simulink model "slexVariantSourceAndSink_org"  (Simulink 10.0)
settings: Solver=FixedStepAuto  StartTime=0.0  StopTime=10.0  RelTol=1e-3  EnableMultiTasking=on
PreLoadFcn:
  | addpath(fileparts(which(bdroot)));
PostLoadFcn:
  | V = Simulink.Parameter(int32(1));
  | V.StorageClass = 'Define (Custom)';
  | V.CoderInfo.CustomAttributes.HeaderFile='variant_defines.h';
  | 
  | W=copy(V);
libraries: simulink x1
settings Model: Creator=The MathWorks, Inc.  LastModifiedBy=bhisma
settings DataIOCC: LimitDataPoints=on  OutputSaveName=out1,out2,out3
settings OptimizationCC: LifeSpan=1  EfficientTunableParamExpr=on
settings DebuggingCC: UnderspecifiedInitializationDetection=Simplified  MergeDetectMultiDrivingBlocksExec=error  ParameterPrecisionLossMsg=none  AllowSymbolicDim=off
settings SFSimCC: MATLABDynamicMemAlloc=off
settings RTWCC: Description=Embedded Coder  SystemTargetFile=ert.tlc  TemplateMakefile=ert_default_tmf
settings CodeAppCC: IgnoreCustomStorageClasses=off  CustomSymbolStrModelFcn=$N
settings ERTTargetCC: MultiwordLength=2048  GenerateSampleERTMain=on  ERTCustomFileTemplate=example_file_process.tlc  ConvertIfToSwitch=off  SuppressUnreachableDefaultCases=off
settings ConfigComp: CovExternalEMLEnable=off

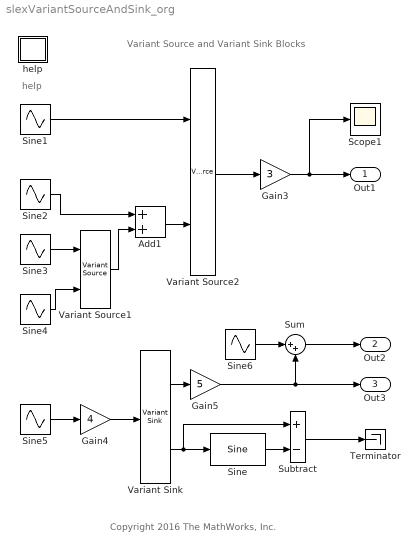
== system slexVariantSourceAndSink_org ==
  note: Variant Source and Variant Sink Blocks
  note: Copyright 2016 The MathWorks, Inc.
  note: help
  Add1 : Sum
  Gain3 : Gain  Gain=3
  Gain4 : Gain  Gain=4
  Gain5 : Gain  Gain=5
  Scope1 : Scope
  Sine : simulink/Lookup Tables/Sine  Formula=sin(2*pi*u)  NumDataPoints=(2^5)+1  OutputWordLength=16  InternalRulePriority=Speed
      settings: SourceProductName=Simulink
  Sine{1..6} (6 alike) : Sin  SineType=Sample based  SampleTime=0.2
  Subtract : Sum  Inputs=+-
  Sum : Sum  Inputs=|++
  Terminator : Terminator
  Variant Sink : VariantSink  VariantControls=DataTag0
      settings: GeneratePreprocessorConditionals=on
  Variant Source1 : VariantSource  VariantControls=DataTag1
  Variant Source2 : VariantSource  VariantControls=DataTag2
      settings: GeneratePreprocessorConditionals=on  AllowZeroVariantControls=on
  help : Subsystem
      mask Display: disp('?')
  Out1 : Outport  VectorParamsAs1DForOutWhenUnconnected=off
  Out2 : Outport  Port=2  VectorParamsAs1DForOutWhenUnconnected=off
  Out3 : Outport  Port=3  VectorParamsAs1DForOutWhenUnconnected=off
  wires:
  Sine1/1 -> Variant Source2/1
  Add1/1 -> Variant Source2/2
  Sine2/1 -> Add1/1
  Variant Source2/1 -> Gain3/1
  Gain3/1 -> Scope1/1, Out1/1
  Gain4/1 -> Variant Sink/1
  Sine5/1 -> Gain4/1
  Sum/1 -> Out2/1
  Variant Sink/1 -> Gain5/1
  Sine6/1 -> Sum/1
  Sine3/1 -> Variant Source1/1
  Sine4/1 -> Variant Source1/2
  Variant Source1/1 -> Add1/2
  Variant Sink/2 -> Subtract/1, Sine/1
  Subtract/1 -> Terminator/1
  Sine/1 -> Subtract/2
  Gain5/1 -> Out3/1, Sum/2

== system slexVariantSourceAndSink_org/help ==
  note: This illustrates how the Variant Source and Sink blocks define variant choice regions based on block connectivity. The variant regions are computed by Simulink when you run " Simulation -> Update Diagram ". The process of computing the variant choice regions is called variant condition propagation. The Variant Source provides variation on the source of a signal and the Variant Sink block provides variation on the destination (sink) of a signal. You can select "Display > Blocks > Variant Conditions" to view the variant condition annotations with a legend as described below.
      |
      | For example, Variant Source1 has conditions W==1 and W==2 for its input ports. W is a variant control variable and is defined in the PostLoadFcn of "File -> Model Properties -> Callbacks". The Sine3 block is active when W==1 and the Sine4 block is active when W==2. Examining the Variant Source2 block, we have the first input port active when V==1 and the second input port active when V==2. The Add1 block is active when V==2 and the propagation continues, when means the Variant Source1 is active when V==2, likewise the Sine3 and Sine4 can only be active when V==2, therefore the Sine3 is assigned the variant condition V==2 && W==1 and the Sine4 is assigned V==2 && W==2.
      |
      | If we select the " Allow zero active variant controls " on the Variant Source2 block parameter dialog , then the Gain3, Scope1, and Out1 will be assigned the variant condition, "V==1 || V==2".
      |
      | The Variant Sink specifies conditions W==1 and W==2 for its output ports. These conditions are propagated forward to the connected blocks. The Gain5 block is assigned the condition, W==1. The Sum block illustrates two key concepts in variant condition propagation:
      | Signals are only variant if explicitly marked or when all paths can be proven to be variant. To make the Sine6, Sum, Out2 variant you need to place a Single-Input Single-Output Variant Source before Out2 (or after Sine6)
      | Reading an inactive signal is equivalent to reading "ground". When W ~= 1, then the bottom input to the Sum block is inactive and Out2 = Sine6 + ground.
      |
      | The second output port of the Variant Sink block has the condition W==2 and this is propagated forward to the Sine, Subtract, and Out4 blocks. If you select " Allow zero active variant controls " on the Variant Sink block parameter dialog , then the Sine5 and Gain4 will be assigned the variant condition W==2.
      |
      | The Variant Source and Variant Sink block have the 'Analyze all choices during update diagram and generate preprocessor conditionals" parameter selected. This means that the generated code from the Simulink Embedded Coder will have #if COND present in the generated code and you select the active choice at code compile-time. If you unselect this parameter, then the generated code will have only the active choice present.
      |
      | Legend
      |
      | To view variant condition annotations for this model, from the Simulink editor menu, select
      | "Display > Blocks > Variant Conditions".
      | If it is already selected, you can run Updated Diagram (^D) to compile the model and display the conditions. There is also a separate Variant Condition legend window.
      | The Variant Condition legend displays on the block " v:C " where C represents the variant condition index on the legend.
      | There are no annotations on unconditional blocks.
      | The v:C labels in the legend are hyper-linked and highlight the blocks with condition, C.
      | The condition in the Description field of the annotation wraps (uses multiple lines when it is long).
      | The table shows the final propagated (computed) conditions for blocks. For example, conditions that you entered in Variant Source blocks may or may not appear in the table. They will only appear in the table if the condition was actually applied to a block. This reduces clutter in the legend.
      | The conditions in the table are sorted.
      | Conditions will be false if the Simulink variant condition expression engine can prove the blocks will never run. For example, Sine4 feeds the 2nd input of Variant Source1. If we change the condition of the 2nd input port on the Variant Source1 dialog, from W==2 to V==4 , this will result in the condition V==4 && V==2 for Sine4 which is always false. This condition arises because the Variant Source1 feeds the Add1 block which is connected to the 2nd input of Variant Source2, which says Variant Source1 will only be active when V==2, therefore Sine4 can only be active when V==4 && V==2 which is always false.
